simulink model "FFM_Punch"  (R2017a)
settings: Solver=ode3  StartTime=0.0  StopTime=timesteps  FixedStep=data.SIM.Ts  RelTol=1e-3  EnableMultiTasking=on
values from neighbouring files (symbols this model uses):
  data =     [dakota_config.mat]
  downshift_map = data.TCU.upshift.veh_spd_default    [Simulation_results.m]
  upshift_map = data.TCU.upshift.veh_spd_default    [Simulation_results.m]
undefined symbols (not defined in the file or in its folder): air_density, Cd, DiscIntNeverNeededParam, fr_crankshaft, fr_speed_values, g, i_FD, ICE, Low_Ratio, M_Eng_Max, M_Eng_Max_Max, M_Eng_Max_Rpm, mt2m_f, mu_Roll_C0, mu_Roll_C1, mu_Roll_C2, Mv, n_Idle_Eng, Overdrive_Ratio, Re, S_eff_drag, Ts
(part 13 of 15)

== system FFM_Punch/Driver Interface/Driver Mode_pedalbased/Driver PID Error Calculation and ffwd/Throttle_Pedal_Determination/Saturation1 ==
  UL : Inport  Tag=Controls_Lib_V1.0  OutDataTypeStr=single  Interpolate=off
  Input : Inport  Tag=Controls_Lib_V1.0  Port=2  OutDataTypeStr=single  Interpolate=off
  LL : Inport  Tag=Controls_Lib_V1.0  Port=3  OutDataTypeStr=single  Interpolate=off
  Logic : Logic  Tag=Controls_Lib  Description=Logic  Operator=OR  Inputs=Inputs  OutDataTypeStr=boolean  SampleTime=SampleTime  mask(Logic){Operator=OR, Inputs=2, IconShape=rectangular, SampleTime=-1, AllPortsSameDT=on, OutDataTypeStr=boolean}
      mask prompts: Inputs "Number of input ports:"; IconShape "Icon shape:"; SampleTime "Sample time (-1 for inherited):"; AllPortsSameDT "Require all inputs and output to have the same data type"; OutDataTypeStr "Output data type:"
      mask help: Logical operators. For a single input, operators are applied across the input vector. For multiple inputs, operators are applied across the inputs.
      mask Help: web([fileparts(which('Lib_built')) filesep 'hlp' filesep 'lib_Logic' '.html'], '-helpbrowser')
      mask TypeOptions Operator: Operator
      mask TypeOptions Inputs: Inputs
      mask TypeOptions IconShape: IconShape
      mask TypeOptions SampleTime: SampleTime
      mask TypeOptions AllPortsSameDT: AllPortsSameDT
      mask TypeOptions OutDataTypeStr: OutDataTypeStr
  MinMax1 : MinMax  Tag=Controls_Lib  Description=MinMax  RequirementInfo={} %GIDa_80f364b9_0622_4713_99d7_f33b776e02e8  Function=max  Inputs=Inputs  OutMin=OutMin  OutMax=OutMax  OutDataTypeStr=single  RndMeth=Zero  SampleTime=SampleTime  InputSameDT=on  mask(MinMax){Function=max, Inputs=2, ZeroCross=on, SampleTime=-1, InputSameDT=on, OutMin=[], OutMax=[], OutDataTypeStr=single, LockScale=off, RndMeth=Zero, SaturateOnIntegerOverflow=off}
      mask prompts: Inputs "Number of input ports:"; ZeroCross "Enable zero-crossing detection"; SampleTime "Sample time (-1 for inherited):"; InputSameDT "Require all inputs to have the same data type"; OutMin "Output minimum:"; OutMax "Output maximum:"; OutDataTypeStr "Output data type:"; LockScale "Lock output data type setting against changes by the fixed-point tools"; RndMeth "Integer rounding mode:"; SaturateOnIntegerOverflow "Saturate on integer overflow"
      mask help: Output min or max of input. For a single input, operators are applied across the input vector. For multiple inputs, operators are applied across the inputs.
      mask Help: web([fileparts(which('Lib_built')) filesep 'hlp' filesep 'lib_MinMax' '.html'], '-helpbrowser')
      mask TypeOptions Function: Function
      mask TypeOptions Inputs: Inputs
      mask TypeOptions ZeroCross: ZeroCross
      mask TypeOptions SampleTime: SampleTime
      mask TypeOptions InputSameDT: InputSameDT
      mask TypeOptions OutMin: OutMin
      mask TypeOptions OutMax: OutMax
      mask TypeOptions OutDataTypeStr: OutDataTypeStr
      mask TypeOptions LockScale: LockScale
      mask TypeOptions RndMeth: RndMeth
      mask TypeOptions SaturateOnIntegerOverflow: SaturateOnIntegerOverflow
  MinMax2 : MinMax  Tag=Controls_Lib  Description=MinMax  RequirementInfo={} %GIDa_7a1d9ff7_0836_420d_85fa_739f6ecc8fec  Inputs=Inputs  OutMin=OutMin  OutMax=OutMax  OutDataTypeStr=single  RndMeth=Zero  SampleTime=SampleTime  InputSameDT=on  mask(MinMax){Function=min, Inputs=2, ZeroCross=on, SampleTime=-1, InputSameDT=on, OutMin=[], OutMax=[], OutDataTypeStr=single, LockScale=off, RndMeth=Zero, SaturateOnIntegerOverflow=off}
      mask prompts: Inputs "Number of input ports:"; ZeroCross "Enable zero-crossing detection"; SampleTime "Sample time (-1 for inherited):"; InputSameDT "Require all inputs to have the same data type"; OutMin "Output minimum:"; OutMax "Output maximum:"; OutDataTypeStr "Output data type:"; LockScale "Lock output data type setting against changes by the fixed-point tools"; RndMeth "Integer rounding mode:"; SaturateOnIntegerOverflow "Saturate on integer overflow"
      mask help: Output min or max of input. For a single input, operators are applied across the input vector. For multiple inputs, operators are applied across the inputs.
      mask Help: web([fileparts(which('Lib_built')) filesep 'hlp' filesep 'lib_MinMax' '.html'], '-helpbrowser')
      mask TypeOptions Function: Function
      mask TypeOptions Inputs: Inputs
      mask TypeOptions ZeroCross: ZeroCross
      mask TypeOptions SampleTime: SampleTime
      mask TypeOptions InputSameDT: InputSameDT
      mask TypeOptions OutMin: OutMin
      mask TypeOptions OutMax: OutMax
      mask TypeOptions OutDataTypeStr: OutDataTypeStr
      mask TypeOptions LockScale: LockScale
      mask TypeOptions RndMeth: RndMeth
      mask TypeOptions SaturateOnIntegerOverflow: SaturateOnIntegerOverflow
  RelationalOperator : RelationalOperator  Tag=Controls_Lib  Description=RelationalOperator  Operator=<  OutDataTypeStr=boolean  SampleTime=SampleTime  RndMeth=Nearest  InputSameDT=on  mask(Relational operator){Operator=<, ZeroCross=on, SampleTime=-1, InputSameDT=on, OutDataTypeStr=boolean}
      mask prompts: Operator "Relational operator:"; ZeroCross "Enable zero-crossing detection"; SampleTime "Sample time (-1 for inherited):"; InputSameDT "Require all inputs to have the same data type"; OutDataTypeStr "Output data type:"
      mask help: Applies the selected relational operator to the inputs and outputs the result. The top (or left) input corresponds to the first operand.
      mask Help: web([fileparts(which('Lib_built')) filesep 'hlp' filesep 'lib_Relational' '.html'], '-helpbrowser')
      mask TypeOptions Operator: Operator
      mask TypeOptions ZeroCross: ZeroCross
      mask TypeOptions SampleTime: SampleTime
      mask TypeOptions InputSameDT: InputSameDT
      mask TypeOptions OutDataTypeStr: OutDataTypeStr
  RelationalOperator1 : RelationalOperator  Tag=Controls_Lib  Description=RelationalOperator  Operator=>  OutDataTypeStr=boolean  SampleTime=SampleTime  RndMeth=Nearest  InputSameDT=on  mask(Relational operator){Operator=>, ZeroCross=on, SampleTime=-1, InputSameDT=on, OutDataTypeStr=boolean}
      mask prompts: Operator "Relational operator:"; ZeroCross "Enable zero-crossing detection"; SampleTime "Sample time (-1 for inherited):"; InputSameDT "Require all inputs to have the same data type"; OutDataTypeStr "Output data type:"
      mask help: Applies the selected relational operator to the inputs and outputs the result. The top (or left) input corresponds to the first operand.
      mask Help: web([fileparts(which('Lib_built')) filesep 'hlp' filesep 'lib_Relational' '.html'], '-helpbrowser')
      mask TypeOptions Operator: Operator
      mask TypeOptions ZeroCross: ZeroCross
      mask TypeOptions SampleTime: SampleTime
      mask TypeOptions InputSameDT: InputSameDT
      mask TypeOptions OutDataTypeStr: OutDataTypeStr
  Output : Outport  Tag=Controls_Lib_V1.0  RequirementInfo={} %GIDa_9fd5db7c_4dee_4852_b779_4842f3ca1f9d  OutDataTypeStr=single  InitialOutput=0
  b_OutpSaturated : Outport  Tag=Controls_Lib_V1.0  RequirementInfo={} %GIDa_d09f5f3b_3dd2_4a13_ad7b_0114fc5d08dd  Port=2  OutDataTypeStr=boolean  InitialOutput=0
  wires:
  Logic/1 -> b_OutpSaturated/1
  MinMax1/1 -> Output/1, RelationalOperator1/1
  LL/1 -> MinMax1/1
  MinMax2/1 -> MinMax1/2, RelationalOperator/1
  Input/1 -> [Input], RelationalOperator/2, MinMax2/2
  UL/1 -> MinMax2/1
  RelationalOperator/1 -> Logic/2
  [Input] -> RelationalOperator1/2
  RelationalOperator1/1 -> Logic/1

== system FFM_Punch/Driver Interface/Driver Mode_pedalbased/Final PID Computation/PIDController/Saturation ==
  UL : Inport  Tag=Controls_Lib_V1.0  OutDataTypeStr=single  Interpolate=off
  Input : Inport  Tag=Controls_Lib_V1.0  Port=2  OutDataTypeStr=single  Interpolate=off
  LL : Inport  Tag=Controls_Lib_V1.0  Port=3  OutDataTypeStr=single  Interpolate=off
  Logic : Logic  Tag=Controls_Lib  Description=Logic  Operator=OR  Inputs=Inputs  OutDataTypeStr=boolean  SampleTime=SampleTime  mask(Logic){Operator=OR, Inputs=2, IconShape=rectangular, SampleTime=-1, AllPortsSameDT=on, OutDataTypeStr=boolean}
      mask prompts: Inputs "Number of input ports:"; IconShape "Icon shape:"; SampleTime "Sample time (-1 for inherited):"; AllPortsSameDT "Require all inputs and output to have the same data type"; OutDataTypeStr "Output data type:"
      mask help: Logical operators. For a single input, operators are applied across the input vector. For multiple inputs, operators are applied across the inputs.
      mask Help: web([fileparts(which('Lib_built')) filesep 'hlp' filesep 'lib_Logic' '.html'], '-helpbrowser')
      mask TypeOptions Operator: Operator
      mask TypeOptions Inputs: Inputs
      mask TypeOptions IconShape: IconShape
      mask TypeOptions SampleTime: SampleTime
      mask TypeOptions AllPortsSameDT: AllPortsSameDT
      mask TypeOptions OutDataTypeStr: OutDataTypeStr
  MinMax1 : MinMax  Tag=Controls_Lib  Description=MinMax  RequirementInfo={} %GIDa_80f364b9_0622_4713_99d7_f33b776e02e8  Function=max  Inputs=Inputs  OutMin=OutMin  OutMax=OutMax  OutDataTypeStr=single  RndMeth=Zero  SampleTime=SampleTime  InputSameDT=on  mask(MinMax){Function=max, Inputs=2, ZeroCross=on, SampleTime=-1, InputSameDT=on, OutMin=[], OutMax=[], OutDataTypeStr=single, LockScale=off, RndMeth=Zero, SaturateOnIntegerOverflow=off}
      mask prompts: Inputs "Number of input ports:"; ZeroCross "Enable zero-crossing detection"; SampleTime "Sample time (-1 for inherited):"; InputSameDT "Require all inputs to have the same data type"; OutMin "Output minimum:"; OutMax "Output maximum:"; OutDataTypeStr "Output data type:"; LockScale "Lock output data type setting against changes by the fixed-point tools"; RndMeth "Integer rounding mode:"; SaturateOnIntegerOverflow "Saturate on integer overflow"
      mask help: Output min or max of input. For a single input, operators are applied across the input vector. For multiple inputs, operators are applied across the inputs.
      mask Help: web([fileparts(which('Lib_built')) filesep 'hlp' filesep 'lib_MinMax' '.html'], '-helpbrowser')
      mask TypeOptions Function: Function
      mask TypeOptions Inputs: Inputs
      mask TypeOptions ZeroCross: ZeroCross
      mask TypeOptions SampleTime: SampleTime
      mask TypeOptions InputSameDT: InputSameDT
      mask TypeOptions OutMin: OutMin
      mask TypeOptions OutMax: OutMax
      mask TypeOptions OutDataTypeStr: OutDataTypeStr
      mask TypeOptions LockScale: LockScale
      mask TypeOptions RndMeth: RndMeth
      mask TypeOptions SaturateOnIntegerOverflow: SaturateOnIntegerOverflow
  MinMax2 : MinMax  Tag=Controls_Lib  Description=MinMax  RequirementInfo={} %GIDa_7a1d9ff7_0836_420d_85fa_739f6ecc8fec  Inputs=Inputs  OutMin=OutMin  OutMax=OutMax  OutDataTypeStr=single  RndMeth=Zero  SampleTime=SampleTime  InputSameDT=on  mask(MinMax){Function=min, Inputs=2, ZeroCross=on, SampleTime=-1, InputSameDT=on, OutMin=[], OutMax=[], OutDataTypeStr=single, LockScale=off, RndMeth=Zero, SaturateOnIntegerOverflow=off}
      mask prompts: Inputs "Number of input ports:"; ZeroCross "Enable zero-crossing detection"; SampleTime "Sample time (-1 for inherited):"; InputSameDT "Require all inputs to have the same data type"; OutMin "Output minimum:"; OutMax "Output maximum:"; OutDataTypeStr "Output data type:"; LockScale "Lock output data type setting against changes by the fixed-point tools"; RndMeth "Integer rounding mode:"; SaturateOnIntegerOverflow "Saturate on integer overflow"
      mask help: Output min or max of input. For a single input, operators are applied across the input vector. For multiple inputs, operators are applied across the inputs.
      mask Help: web([fileparts(which('Lib_built')) filesep 'hlp' filesep 'lib_MinMax' '.html'], '-helpbrowser')
      mask TypeOptions Function: Function
      mask TypeOptions Inputs: Inputs
      mask TypeOptions ZeroCross: ZeroCross
      mask TypeOptions SampleTime: SampleTime
      mask TypeOptions InputSameDT: InputSameDT
      mask TypeOptions OutMin: OutMin
      mask TypeOptions OutMax: OutMax
      mask TypeOptions OutDataTypeStr: OutDataTypeStr
      mask TypeOptions LockScale: LockScale
      mask TypeOptions RndMeth: RndMeth
      mask TypeOptions SaturateOnIntegerOverflow: SaturateOnIntegerOverflow
  RelationalOperator : RelationalOperator  Tag=Controls_Lib  Description=RelationalOperator  Operator=<  OutDataTypeStr=boolean  SampleTime=SampleTime  RndMeth=Nearest  InputSameDT=on  mask(Relational operator){Operator=<, ZeroCross=on, SampleTime=-1, InputSameDT=on, OutDataTypeStr=boolean}
      mask prompts: Operator "Relational operator:"; ZeroCross "Enable zero-crossing detection"; SampleTime "Sample time (-1 for inherited):"; InputSameDT "Require all inputs to have the same data type"; OutDataTypeStr "Output data type:"
      mask help: Applies the selected relational operator to the inputs and outputs the result. The top (or left) input corresponds to the first operand.
      mask Help: web([fileparts(which('Lib_built')) filesep 'hlp' filesep 'lib_Relational' '.html'], '-helpbrowser')
      mask TypeOptions Operator: Operator
      mask TypeOptions ZeroCross: ZeroCross
      mask TypeOptions SampleTime: SampleTime
      mask TypeOptions InputSameDT: InputSameDT
      mask TypeOptions OutDataTypeStr: OutDataTypeStr
  RelationalOperator1 : RelationalOperator  Tag=Controls_Lib  Description=RelationalOperator  Operator=>  OutDataTypeStr=boolean  SampleTime=SampleTime  RndMeth=Nearest  InputSameDT=on  mask(Relational operator){Operator=>, ZeroCross=on, SampleTime=-1, InputSameDT=on, OutDataTypeStr=boolean}
      mask prompts: Operator "Relational operator:"; ZeroCross "Enable zero-crossing detection"; SampleTime "Sample time (-1 for inherited):"; InputSameDT "Require all inputs to have the same data type"; OutDataTypeStr "Output data type:"
      mask help: Applies the selected relational operator to the inputs and outputs the result. The top (or left) input corresponds to the first operand.
      mask Help: web([fileparts(which('Lib_built')) filesep 'hlp' filesep 'lib_Relational' '.html'], '-helpbrowser')
      mask TypeOptions Operator: Operator
      mask TypeOptions ZeroCross: ZeroCross
      mask TypeOptions SampleTime: SampleTime
      mask TypeOptions InputSameDT: InputSameDT
      mask TypeOptions OutDataTypeStr: OutDataTypeStr
  Output : Outport  Tag=Controls_Lib_V1.0  RequirementInfo={} %GIDa_9fd5db7c_4dee_4852_b779_4842f3ca1f9d  OutDataTypeStr=single  InitialOutput=0
  b_OutpSaturated : Outport  Tag=Controls_Lib_V1.0  RequirementInfo={} %GIDa_d09f5f3b_3dd2_4a13_ad7b_0114fc5d08dd  Port=2  OutDataTypeStr=boolean  InitialOutput=0
  wires:
  Logic/1 -> b_OutpSaturated/1
  MinMax1/1 -> Output/1, RelationalOperator1/1
  LL/1 -> MinMax1/1
  MinMax2/1 -> MinMax1/2, RelationalOperator/1
  Input/1 -> [Input], RelationalOperator/2, MinMax2/2
  UL/1 -> MinMax2/1
  RelationalOperator/1 -> Logic/2
  [Input] -> RelationalOperator1/2
  RelationalOperator1/1 -> Logic/1

== system FFM_Punch/Driver Interface/Driver Mode_pedalbased/Final PID Computation/PIDController/Saturation1 ==
  UL : Inport  Tag=Controls_Lib_V1.0  OutDataTypeStr=single  Interpolate=off
  Input : Inport  Tag=Controls_Lib_V1.0  Port=2  OutDataTypeStr=single  Interpolate=off
  LL : Inport  Tag=Controls_Lib_V1.0  Port=3  OutDataTypeStr=single  Interpolate=off
  Logic : Logic  Tag=Controls_Lib  Description=Logic  Operator=OR  Inputs=Inputs  OutDataTypeStr=boolean  SampleTime=SampleTime  mask(Logic){Operator=OR, Inputs=2, IconShape=rectangular, SampleTime=-1, AllPortsSameDT=on, OutDataTypeStr=boolean}
      mask prompts: Inputs "Number of input ports:"; IconShape "Icon shape:"; SampleTime "Sample time (-1 for inherited):"; AllPortsSameDT "Require all inputs and output to have the same data type"; OutDataTypeStr "Output data type:"
      mask help: Logical operators. For a single input, operators are applied across the input vector. For multiple inputs, operators are applied across the inputs.
      mask Help: web([fileparts(which('Lib_built')) filesep 'hlp' filesep 'lib_Logic' '.html'], '-helpbrowser')
      mask TypeOptions Operator: Operator
      mask TypeOptions Inputs: Inputs
      mask TypeOptions IconShape: IconShape
      mask TypeOptions SampleTime: SampleTime
      mask TypeOptions AllPortsSameDT: AllPortsSameDT
      mask TypeOptions OutDataTypeStr: OutDataTypeStr
  MinMax1 : MinMax  Tag=Controls_Lib  Description=MinMax  RequirementInfo={} %GIDa_80f364b9_0622_4713_99d7_f33b776e02e8  Function=max  Inputs=Inputs  OutMin=OutMin  OutMax=OutMax  OutDataTypeStr=single  RndMeth=Zero  SampleTime=SampleTime  InputSameDT=on  mask(MinMax){Function=max, Inputs=2, ZeroCross=on, SampleTime=-1, InputSameDT=on, OutMin=[], OutMax=[], OutDataTypeStr=single, LockScale=off, RndMeth=Zero, SaturateOnIntegerOverflow=off}
      mask prompts: Inputs "Number of input ports:"; ZeroCross "Enable zero-crossing detection"; SampleTime "Sample time (-1 for inherited):"; InputSameDT "Require all inputs to have the same data type"; OutMin "Output minimum:"; OutMax "Output maximum:"; OutDataTypeStr "Output data type:"; LockScale "Lock output data type setting against changes by the fixed-point tools"; RndMeth "Integer rounding mode:"; SaturateOnIntegerOverflow "Saturate on integer overflow"
      mask help: Output min or max of input. For a single input, operators are applied across the input vector. For multiple inputs, operators are applied across the inputs.
      mask Help: web([fileparts(which('Lib_built')) filesep 'hlp' filesep 'lib_MinMax' '.html'], '-helpbrowser')
      mask TypeOptions Function: Function
      mask TypeOptions Inputs: Inputs
      mask TypeOptions ZeroCross: ZeroCross
      mask TypeOptions SampleTime: SampleTime
      mask TypeOptions InputSameDT: InputSameDT
      mask TypeOptions OutMin: OutMin
      mask TypeOptions OutMax: OutMax
      mask TypeOptions OutDataTypeStr: OutDataTypeStr
      mask TypeOptions LockScale: LockScale
      mask TypeOptions RndMeth: RndMeth
      mask TypeOptions SaturateOnIntegerOverflow: SaturateOnIntegerOverflow
  MinMax2 : MinMax  Tag=Controls_Lib  Description=MinMax  RequirementInfo={} %GIDa_7a1d9ff7_0836_420d_85fa_739f6ecc8fec  Inputs=Inputs  OutMin=OutMin  OutMax=OutMax  OutDataTypeStr=single  RndMeth=Zero  SampleTime=SampleTime  InputSameDT=on  mask(MinMax){Function=min, Inputs=2, ZeroCross=on, SampleTime=-1, InputSameDT=on, OutMin=[], OutMax=[], OutDataTypeStr=single, LockScale=off, RndMeth=Zero, SaturateOnIntegerOverflow=off}
      mask prompts: Inputs "Number of input ports:"; ZeroCross "Enable zero-crossing detection"; SampleTime "Sample time (-1 for inherited):"; InputSameDT "Require all inputs to have the same data type"; OutMin "Output minimum:"; OutMax "Output maximum:"; OutDataTypeStr "Output data type:"; LockScale "Lock output data type setting against changes by the fixed-point tools"; RndMeth "Integer rounding mode:"; SaturateOnIntegerOverflow "Saturate on integer overflow"
      mask help: Output min or max of input. For a single input, operators are applied across the input vector. For multiple inputs, operators are applied across the inputs.
      mask Help: web([fileparts(which('Lib_built')) filesep 'hlp' filesep 'lib_MinMax' '.html'], '-helpbrowser')
      mask TypeOptions Function: Function
      mask TypeOptions Inputs: Inputs
      mask TypeOptions ZeroCross: ZeroCross
      mask TypeOptions SampleTime: SampleTime
      mask TypeOptions InputSameDT: InputSameDT
      mask TypeOptions OutMin: OutMin
      mask TypeOptions OutMax: OutMax
      mask TypeOptions OutDataTypeStr: OutDataTypeStr
      mask TypeOptions LockScale: LockScale
      mask TypeOptions RndMeth: RndMeth
      mask TypeOptions SaturateOnIntegerOverflow: SaturateOnIntegerOverflow
  RelationalOperator : RelationalOperator  Tag=Controls_Lib  Description=RelationalOperator  Operator=<  OutDataTypeStr=boolean  SampleTime=SampleTime  RndMeth=Nearest  InputSameDT=on  mask(Relational operator){Operator=<, ZeroCross=on, SampleTime=-1, InputSameDT=on, OutDataTypeStr=boolean}
      mask prompts: Operator "Relational operator:"; ZeroCross "Enable zero-crossing detection"; SampleTime "Sample time (-1 for inherited):"; InputSameDT "Require all inputs to have the same data type"; OutDataTypeStr "Output data type:"
      mask help: Applies the selected relational operator to the inputs and outputs the result. The top (or left) input corresponds to the first operand.
      mask Help: web([fileparts(which('Lib_built')) filesep 'hlp' filesep 'lib_Relational' '.html'], '-helpbrowser')
      mask TypeOptions Operator: Operator
      mask TypeOptions ZeroCross: ZeroCross
      mask TypeOptions SampleTime: SampleTime
      mask TypeOptions InputSameDT: InputSameDT
      mask TypeOptions OutDataTypeStr: OutDataTypeStr
  RelationalOperator1 : RelationalOperator  Tag=Controls_Lib  Description=RelationalOperator  Operator=>  OutDataTypeStr=boolean  SampleTime=SampleTime  RndMeth=Nearest  InputSameDT=on  mask(Relational operator){Operator=>, ZeroCross=on, SampleTime=-1, InputSameDT=on, OutDataTypeStr=boolean}
      mask prompts: Operator "Relational operator:"; ZeroCross "Enable zero-crossing detection"; SampleTime "Sample time (-1 for inherited):"; InputSameDT "Require all inputs to have the same data type"; OutDataTypeStr "Output data type:"
      mask help: Applies the selected relational operator to the inputs and outputs the result. The top (or left) input corresponds to the first operand.
      mask Help: web([fileparts(which('Lib_built')) filesep 'hlp' filesep 'lib_Relational' '.html'], '-helpbrowser')
      mask TypeOptions Operator: Operator
      mask TypeOptions ZeroCross: ZeroCross
      mask TypeOptions SampleTime: SampleTime
      mask TypeOptions InputSameDT: InputSameDT
      mask TypeOptions OutDataTypeStr: OutDataTypeStr
  Output : Outport  Tag=Controls_Lib_V1.0  RequirementInfo={} %GIDa_9fd5db7c_4dee_4852_b779_4842f3ca1f9d  OutDataTypeStr=single  InitialOutput=0
  b_OutpSaturated : Outport  Tag=Controls_Lib_V1.0  RequirementInfo={} %GIDa_d09f5f3b_3dd2_4a13_ad7b_0114fc5d08dd  Port=2  OutDataTypeStr=boolean  InitialOutput=0
  wires:
  Logic/1 -> b_OutpSaturated/1
  MinMax1/1 -> Output/1, RelationalOperator1/1
  LL/1 -> MinMax1/1
  MinMax2/1 -> MinMax1/2, RelationalOperator/1
  Input/1 -> [Input], RelationalOperator/2, MinMax2/2
  UL/1 -> MinMax2/1
  RelationalOperator/1 -> Logic/2
  [Input] -> RelationalOperator1/2
  RelationalOperator1/1 -> Logic/1

== system FFM_Punch/Driver Interface/Driver Model/Driver Pedals Determination/Brake_Pedal_Determination/Saturation Dynamic ==
  up : Inport
  u : Inport  Port=2
  lo : Inport  Port=3
  Data Type Duplicate : DataTypeDuplicate  DisableCoverage=on
  Data Type Propagation : S-Function  FunctionName=sfix_dtprop  Parameters=14,PropDataTypeMode,(getdatatypespecs(PropDataType,PropScaling,DblOver,0, 0, PropDataTypeMode, PropScalingMode)),IfRefDouble,IfRefSingle,IsSigned,NumBitsBase,NumBitsMult,NumBitsAdd,(sort(reshape(round(NumBitsAllowFinal), prod(size(NumBitsAllowFinal)),1))),PropScalingMode,ValuesUsedBestPrec,SlopeBase,SlopeMult,SlopeAdd,BiasBase,BiasMult,BiasAdd,DblOver  SFunctionDeploymentMode=off  EnableBusSupport=off  mask(Data Type Propagation){PropDataTypeMode=Specify via dialog, PropDataType=fixdt('single'), IfRefDouble=double, IfRefSingle=single, IsSigned=IsSigned1, NumBitsBase=NumBits1, NumBitsMult=1, NumBitsAdd=0, NumBitsAllowFinal=1:128, PropScalingMode=Specify via dialog, PropScaling=2^-10, ValuesUsedBestPrec=[5 -7], SlopeBase=Slope1, SlopeMult=1, SlopeAdd=0, BiasBase=Bias1, BiasMult=1, BiasAdd=0}
      mask prompts: PropDataTypeMode "Simulink:masks:x1PropagatedDataType_MP"; PropDataType "Simulink:masks:x11PropagatedDataTypeegFixdt116Fixdtsingle_MP"; IfRefDouble "Simulink:masks:x11IfAnyReferenceInputIsDoubleOutputIs_MP"; IfRefSingle "Simulink:masks:x12IfAnyReferenceInputIsSingleOutputIs_MP"; IsSigned "Simulink:masks:x13IsSigned_MP"; NumBitsBase "Simulink:masks:x141NumberofBitsBase_MP"; NumBitsMult "Simulink:masks:x142NumberofBitsMultiplicativeAdjustment_MP"; NumBitsAdd "Simulink:masks:x143NumberofBitsAdditiveAdjustment_MP"; NumBitsAllowFinal "Simulink:masks:x144NumberofBitsAllowableFinalValues_MP"; PropScalingMode "Simulink:masks:x2PropagatedScaling_MP"; PropScaling "Simulink:masks:x21PropagatedScalingSlopeEg29OrSlopeBiasEg1253_MP"; ValuesUsedBestPrec "Simulink:masks:x21ValuesUsedToDetermineBestPrecisionScaling_MP"; SlopeBase "Simulink:masks:x211SlopeBase_MP"; SlopeMult "Simulink:masks:x212SlopeMultiplicativeAdjustment_MP"; SlopeAdd "Simulink:masks:x213SlopeAdditiveAdjustment_MP"; BiasBase "Simulink:masks:x221BiasBase_MP"; BiasMult "Simulink:masks:x222BiasMultiplicativeAdjustment_MP"; BiasAdd "Simulink:masks:x223BiasAdditiveAdjustment_MP"
      mask help: Simulink:masks:DataTypePropagation_MD
      mask init:
      | DblOver = 0;
      mask TypeOptions PropDataTypeMode: Simulink:masks:SpecifyViaDialog | Simulink:masks:InheritViaPropagationRule
      mask Callback PropDataTypeMode: fixptdialog(gcbh)
      mask Callback PropDataType: fixptdialog(gcbh)
      mask TypeOptions IfRefDouble: Simulink:masks:double | Simulink:masks:single
      mask TypeOptions IfRefSingle: Simulink:masks:double | Simulink:masks:single
      mask TypeOptions IsSigned: Simulink:masks:IsSigned1 | Simulink:masks:IsSigned2 | Simulink:masks:IsSigned1OrIsSigned2 | Simulink:masks:TRUE | Simulink:masks:FALSE
      mask TypeOptions NumBitsBase: NumBits1 | NumBits2 | max([NumBits1 NumBits2]) | min([NumBits1 NumBits2]) | NumBits1+NumBits2
      mask TypeOptions PropScalingMode: Simulink:masks:SpecifyViaDialog | Simulink:masks:InheritViaPropagationRule | Simulink:masks:ObtainViaBestPrecision
      mask Callback PropScalingMode: fixptdialog(gcbh)
      mask TypeOptions SlopeBase: Slope1 | Slope2 | max([Slope1 Slope2]) | min([Slope1 Slope2]) | Slope1*Slope2 | Slope1/Slope2 | PosRange1 | PosRange2 | max([PosRange1 PosRange2]) | min([PosRange1 PosRange2]) | PosRange1*PosRange2 | PosRange1/PosRange2
      mask TypeOptions BiasBase: Bias1 | Bias2 | max([Bias1 Bias2]) | min([Bias1 Bias2]) | Bias1*Bias2 | Bias1/Bias2 | Bias1+Bias2 | Bias1-Bias2
      mask Display:
      | port_label('Input',1,'Ref1');
      | port_label('Input',2,'Ref2');
      | port_label('Input',3,'Prop');
  LowerRelop1 : RelationalOperator  DisableCoverage=on  Operator=>  OutDataTypeStr=boolean  RndMeth=Nearest
  Switch : Switch  Criteria=u2 ~= 0  OutDataTypeStr=Inherit: Inherit via back propagation  ZeroCross=off
  Switch2 : Switch  Criteria=u2 ~= 0  OutMin=OutMin  OutMax=OutMax  OutDataTypeStr=Inherit: Inherit via back propagation  ZeroCross=off
  UpperRelop : RelationalOperator  DisableCoverage=on  Operator=<  OutDataTypeStr=boolean  RndMeth=Nearest
  y : Outport  OutMin=OutMin  OutMax=OutMax
  wires:
  up/1 -> Switch2/1, LowerRelop1/2
  u/1 -> Data Type Propagation/2, Data Type Propagation/1, LowerRelop1/1, Switch/3, UpperRelop/1
  lo/1 -> Switch/1, UpperRelop/2
  Switch/1 -> Data Type Duplicate/2, Switch2/3, Data Type Propagation/3
  Switch2/1 -> Data Type Duplicate/1, y/1
  LowerRelop1/1 -> Switch2/2
  UpperRelop/1 -> Switch/2
